simulink model "synchro"  (R2020b)
settings: Solver=VariableStepAuto  StartTime=0.0  StopTime=0.0101  RelTol=1e-3
settings Model: Creator=miguel  LastModifiedBy=miguel

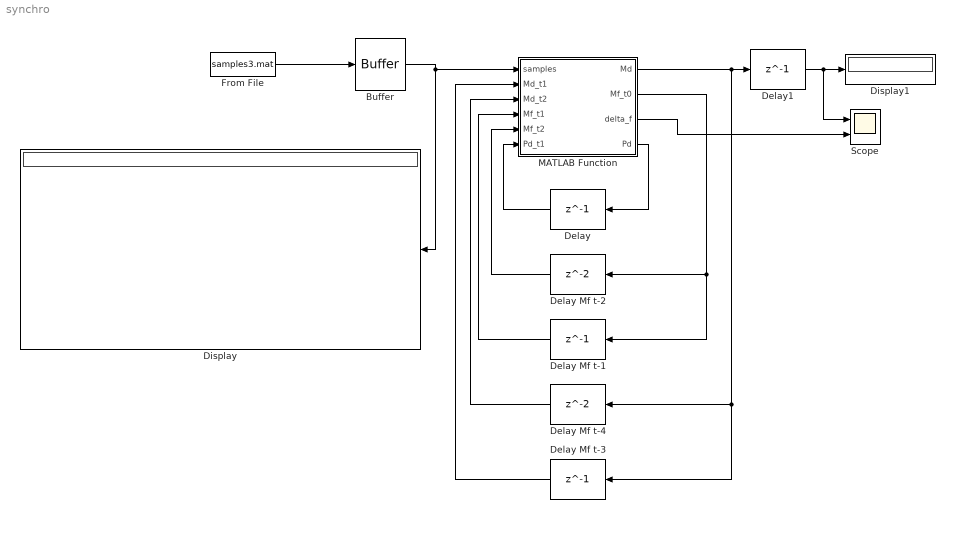
== system synchro ==
  Buffer : Buffer  V=63  OutputFrames=off
  Delay : Delay  DelayLength=1  InputProcessing=Columns as channels (frame based)
  Delay Mf t-1 : Delay  DelayLength=1  InitialCondition=0  UseCircularBuffer=on
  Delay Mf t-2 : Delay  InitialCondition=0  UseCircularBuffer=on
  Delay Mf t-3 : Delay  DelayLength=1  InitialCondition=0  UseCircularBuffer=on
  Delay Mf t-4 : Delay  InitialCondition=0  UseCircularBuffer=on
  Delay1 : Delay  DelayLength=1  InitialCondition=0  UseCircularBuffer=on
  Display : Display
  Display1 : Display
  From File : FromFile  FileName=samples3.mat  SampleTime=50e-9  ExtrapolationAfterLastDataPoint=Ground value
  MATLAB Function : MATLAB Function  TreatAsAtomicUnit=on
  Scope : Scope  NumInputPorts=2
  wires:
  From File/1 -> Buffer/1
  Buffer/1 -> Display/1, MATLAB Function/1(samples)
  Delay Mf t-2/1 -> MATLAB Function/5(Mf_t2)
  Delay Mf t-1/1 -> MATLAB Function/4(Mf_t1)
  MATLAB Function/3(delta_f) -> Scope/2
  MATLAB Function/2(Mf_t0) -> Delay Mf t-2/1, Delay Mf t-1/1
  MATLAB Function/4(Pd) -> Delay/1
  Delay/1 -> MATLAB Function/6(Pd_t1)
  Delay Mf t-3/1 -> MATLAB Function/2(Md_t1)
  Delay Mf t-4/1 -> MATLAB Function/3(Md_t2)
  MATLAB Function/1(Md) -> Delay Mf t-3/1, Delay Mf t-4/1, Delay1/1
  Delay1/1 -> Scope/1, Display1/1

== matlab function synchro/MATLAB Function ==
  data: samples input; Md_t1 input; Md_t2 input; Mf_t1 input; Mf_t2 input; Pd_t1 input; Md output; Mf_t0 output; delta_f output; Pd output
function [Md, Mf_t0, delta_f, Pd]= fcn(samples, Md_t1  , Md_t2 , Mf_t1, Mf_t2, Pd_t1)
% samples of size 64
%#codegen
L = 32;
Ng = 2;

Pd = 0 + 0*i;
Rf = 0;
delta_f = 0;

for m=1:2*L
    if m<=L
        Pd = Pd + samples(m+L) * conj(samples(m));
    end
    Rf = Rf + 0.5 * abs(samples(m))^2;
end
disp(Mf_t2)
Mf_t0 = (abs(Pd)^2)/(Rf^2);
Mf = [Mf_t2 Mf_t1 Mf_t0];
Mf_moy = 0;

for k=1:(Ng+1)
    Mf_moy = Mf_moy + (1/(Ng+1)) * Mf(k);
end

if Mf_moy > 0.8
    if Md_t1 > Md_t2 && Md_t1 > Mf_moy
        phase = angle(Pd_t1);
        delta_f = phase/(pi * 64 * 50e-9);
    end
end

Md = Mf_moy;
